simulink model "rigLoggerMultipacket"  (R2012b)
settings: Solver=FixedStepDiscrete  StartTime=0.0  StopTime=10.0  FixedStep=0.001  RelTol=1e-3
undefined symbols (not defined in the file): macaddr, modelConstants
libraries: simulink x42, xpcethernetlib x29, xpcnetworkbufferlib x15, xpcutilitieslib x14, dspswit3 x14, dspmtrx3 x14, Lib_FileLoggerMultipacket x1
(part 4 of 5)

== matlab function rigLoggerMultipacket/Neural2 Data & Format1/File Logger Format/File Logger Multipacket/Send Multipacket UDP/For Iterator
Subsystem/MATLAB Function ==
  data: data input uint8; numPackets input uint16 size=1; idxPacket input uint16 size=1; packetIP output uint8; lengthIP output uint16 size=1; sourceIP input uint8 size=4; sourcePort input uint16 size=1; destIP input uint8 size=4; destPort input uint16; datagramId input; prependHeader input
function [packetIP, lengthIP] = buildSubPacket(data, numPackets, idxPacket, sourceIP, sourcePort, destIP, destPort, datagramId, prependHeader)
%#codegen
% Creates a single UDP/IP packet that transmits one fragment of a possibly
% multi-fragment set of IP packets carrying the payload in data. idxPacket
% is the index of the fragment to send (1-indexed), out of num packets
% total fragments.
%
% Inputs:  
%   data : uint8 Nx1 or 1xN packet data vectors
%   numPackets, idxPacket : uint16 scalars
%   sourceIP, destIP : 1x4 uint8 of the IP (in address order)
%   sourcePort, destPort : uint16 port numbers
%   datagramId : uint16 scalar, unique id for this set of packets, for this timestep
%    that is used by the receiving IP stack to reassemble fragments
%   prependHeader : uint8 flag determining whether to prepend a 4 byte
%     header containing a 2 byte data length (excluding the header) and a 2
%     byte checksum (sum of bytes modulo 65536) of the data (excluding the 
%     header)
%
% Outputs:
%   packetIP : uint8 1500x1 IP packet to be passed into Create Ethernet
%     Packet block
%   lengthIP : uint16 scalar indicating the total length of packetIP
%     utilized, guaranteed to be even
% 
% Dan O'Shea, Paul Nuyujukian, Vikash Gilja
%

%% Initialize and return early if empty
packetIP = zeros(1500, 1, 'uint8');
lengthIP = uint16(0);

dataLength = numel(data);
if dataLength == 0
    return;
end

%% Build UDP subpacket

packetUDP = zeros(1480, 1, 'uint8');

% 1472 bytes per fragment
bytesPerFragment = uint16(1480);
headerUdpLength = uint16(8);
if prependHeader
    % 6 byte header on first packet containing '#u', 2 byte length, 2 byte checksum
    headerPreLength = uint16(4);
else
    headerPreLength = uint16(0);
end

headerLength = headerPreLength + headerUdpLength;

fragment = zeros(bytesPerFragment, 1, 'uint8');

% slice out the portion of data that goes in this packet
if idxPacket == 1
    byteStart = uint16(1);
    bytesThisFragment = bytesPerFragment - headerLength;
else
    % the first packet only graps 1480-8 bytes
    byteStart = uint16((idxPacket-uint16(1)) * bytesPerFragment - headerLength + uint16(1));
    bytesThisFragment = bytesPerFragment;
end

if byteStart > numel(data)
    % shouldn't happen, means idxPacket was too high for data
    return;
end
byteEnd = byteStart + bytesThisFragment - uint16(1);
% truncate fragment to data length
if byteEnd > numel(data)
    byteEnd = uint16(numel(data));
end
bytesThisFragment = byteEnd - byteStart + 1;

fragment(1:bytesThisFragment) = data(byteStart : byteEnd);

if idxPacket == 1
    if prependHeader
        headerPre = zeros(headerPreLength, 1, 'uint8');
        % 2 byte length
        headerPre(1:2) = typecast(uint16(numel(data)), 'uint8');
        % 2 byte modular checksum
        checksum = uint16(mod(sum(uint32(fragment)), uint32(65536)));
        headerPre(3:4) = typecast(checksum, 'uint8');
    else
        headerPre = [];
    end
        
    % include 8 byte udp header
    headerUdp = zeros(8, 1, 'uint8');
    FFFF = uint16(hex2dec('FFFF'));
    protocol = uint8(hex2dec('11'));
    length_BE = (typecast(uint16(numel(data)) + headerLength, 'uint8')); % flip to big endian
    length_BE = length_BE(end:-1:1);
    sourcePort_BE = (typecast(sourcePort, 'uint8'));
    sourcePort_BE = sourcePort_BE(end:-1:1);
    destPort_BE   = (typecast(destPort,   'uint8'));
    destPort_BE = destPort_BE(end:-1:1);
    headerUdp(1:8) = [sourcePort_BE destPort_BE length_BE uint8([0 0])];
    pseudoHeader = [sourceIP' destIP' uint8(0) protocol length_BE];
    
    if prependHeader
        % include 4 byte header in checksum
        if floor(double(numel(data)) / 2.0) ~= double(numel(data)) / 2.0
            % data is odd length, pad with zero byte
            checksumUdp = FFFF - uint16(mod( uint32(sum( typecast([pseudoHeader headerUdp' headerPre' data(:)' uint8(0)], 'uint16') )), uint32(FFFF) ));
        else
            checksumUdp = FFFF - uint16(mod( uint32(sum( typecast([pseudoHeader headerUdp' headerPre' data(:)'], 'uint16') )), uint32(FFFF) ));
        end
    else
        if floor(double(numel(data)) / 2.0) ~= double(numel(data)) / 2.0
            % data is odd length, pad with zero byte
            checksumUdp = FFFF - uint16(mod( uint32(sum( typecast([pseudoHeader headerUdp' data(:)' uint8(0)], 'uint16') )), uint32(FFFF) ));
        else
            checksumUdp = FFFF - uint16(mod( uint32(sum( typecast([pseudoHeader headerUdp' data(:)'], 'uint16') )), uint32(FFFF) ));
        end
    end
    headerUdp(7:8) = typecast(checksumUdp, 'uint8');

    % include custom 4 byte custom header with length and checksum
    if prependHeader
        lengthUDP = uint16(numel(headerUdp) + numel(headerPre) + bytesThisFragment);
        packetUDP(1:lengthUDP) = [headerUdp; headerPre; fragment(1:bytesThisFragment)];
    else
        % no header
        lengthUDP = uint16(numel(headerUdp) + bytesThisFragment);
        packetUDP(1:lengthUDP) = [headerUdp; fragment(1:bytesThisFragment)];
    end
else
    lengthUDP = uint16(bytesThisFragment);
    packetUDP(1:lengthUDP) = fragment(1:bytesThisFragment);
end

%% Build the fragment information that goes into IP header

% first 3 bits are 0, 1=DF, 2=More Fragments
% next 15 bits are length of fragment in bytes / 8
if idxPacket == 1
    fragmentWord = uint16(0);
else
    fragmentWord = (byteStart - uint16(1) + headerLength) / uint16(8);
end
if idxPacket < numPackets
    % set the more fragments bit
    fragmentWord = bitset(fragmentWord, 14);
end

% swap to big endian
fragmentBytes = typecast(fragmentWord, 'uint8')';
fragmentBytes = fragmentBytes([2;1]);

%% Build IP packet for this fragment

% make udp content length even
if floor(double(lengthUDP) / 2) ~= (double(lengthUDP) / 2)
    lengthUDP = lengthUDP + uint16(1);
end

% build IP header
lengthIP = lengthUDP + uint16(20);
version_IHL = uint8(69); % IPv4 and IP header length of 5
ToS = uint8(0); % no QOS on network

length_BE = (typecast(lengthIP, 'uint8')); % change to big endian
length_BE = length_BE(end:-1:1);

%ff = [ uint8(bin2dec('01000000')) 0 ]; % don't fragment packets
ff = fragmentBytes';
TTL = uint8(10); % ttl to 10 seconds/hops
protocol = uint8(hex2dec('11')); % UDP Protocol
headerIP = [ version_IHL ToS length_BE datagramId' ff TTL protocol 0 0 sourceIP' destIP'];

FFFF = uint16(hex2dec('FFFF'));
checksum = FFFF - uint16(mod( uint32(sum( typecast(headerIP, 'uint16') )), uint32(FFFF) ));
headerIP(11:12) = typecast(checksum, 'uint8');

% assemble the final packet
packetIP(1:lengthIP) = [ headerIP'; packetUDP(1:lengthUDP) ];

== matlab function rigLoggerMultipacket/DecoderC Data & Format1/File Logger Format/File Logger Multipacket/Send Multipacket UDP/For Iterator
Subsystem/MATLAB Function1 ==
  data: idx input; vec output; in input
function vec = storeInVector(idx, in)
%#codegen

nPacketsMax = 15;

persistent pVec;
if isempty(pVec) || idx == 1
    pVec = repmat(in*0, nPacketsMax, 1);
end
if idx >= 1 && idx <= nPacketsMax
    pVec(idx) = in;
end

vec = pVec;

== matlab function rigLoggerMultipacket/DecoderC Data & Format1/File Logger Format/File Logger Multipacket/Send Multipacket UDP/MATLAB Function ==
  data: in input; numPackets output uint16 size=1; prependHeader input
function numPackets = computeNumPackets(in, prependHeader)
%#codegen

% Assuming 1500 MTU, 1480 bytes per IP packet
% 8 bytes in udp header + 4 bytes in custom header if used, but only on the
% first fragment sent
if prependHeader
    headerLength = 8 + 6;
else
    headerLength = 8;
end
numPackets = uint16(ceil((double(numel(in))+headerLength) / 1480));

== matlab function rigLoggerMultipacket/DecoderC Data & Format1/File Logger Format/File Logger Multipacket/Send Multipacket UDP/MATLAB Function1 ==
  data: transmitId input uint8 size=1; datagramId output uint8 size=2
function datagramId = getDatagramId(transmitId)
%#codegen

% generates a unique id for this block, for this packet

persistent pId
if isempty(pId)
    pId = uint8(0);
else
    pId = pId + uint8(1);
end

datagramId = [transmitId; pId];

== matlab function rigLoggerMultipacket/DecoderD Data & Format1/File Logger Data/File Logger Multipacket/MATLAB Function1 ==
  data: u input; y output
function y = padFileName(u)

z = uint8(zeros(20, 1));

z(1:length(u)) = u;

y = z';

== matlab function rigLoggerMultipacket/DecoderD Data & Format1/File Logger Data/File Logger Multipacket/Send Multipacket UDP/For Iterator
Subsystem/MATLAB Function ==
  data: data input uint8; numPackets input uint16 size=1; idxPacket input uint16 size=1; packetIP output uint8; lengthIP output uint16 size=1; sourceIP input uint8 size=4; sourcePort input uint16 size=1; destIP input uint8 size=4; destPort input uint16; datagramId input; prependHeader input
function [packetIP, lengthIP] = buildSubPacket(data, numPackets, idxPacket, sourceIP, sourcePort, destIP, destPort, datagramId, prependHeader)
%#codegen
% Creates a single UDP/IP packet that transmits one fragment of a possibly
% multi-fragment set of IP packets carrying the payload in data. idxPacket
% is the index of the fragment to send (1-indexed), out of num packets
% total fragments.
%
% Inputs:  
%   data : uint8 Nx1 or 1xN packet data vectors
%   numPackets, idxPacket : uint16 scalars
%   sourceIP, destIP : 1x4 uint8 of the IP (in address order)
%   sourcePort, destPort : uint16 port numbers
%   datagramId : uint16 scalar, unique id for this set of packets, for this timestep
%    that is used by the receiving IP stack to reassemble fragments
%   prependHeader : uint8 flag determining whether to prepend a 4 byte
%     header containing a 2 byte data length (excluding the header) and a 2
%     byte checksum (sum of bytes modulo 65536) of the data (excluding the 
%     header)
%
% Outputs:
%   packetIP : uint8 1500x1 IP packet to be passed into Create Ethernet
%     Packet block
%   lengthIP : uint16 scalar indicating the total length of packetIP
%     utilized, guaranteed to be even
% 
% Dan O'Shea, Paul Nuyujukian, Vikash Gilja
%

%% Initialize and return early if empty
packetIP = zeros(1500, 1, 'uint8');
lengthIP = uint16(0);

dataLength = numel(data);
if dataLength == 0
    return;
end

%% Build UDP subpacket

packetUDP = zeros(1480, 1, 'uint8');

% 1472 bytes per fragment
bytesPerFragment = uint16(1480);
headerUdpLength = uint16(8);
if prependHeader
    % 6 byte header on first packet containing '#u', 2 byte length, 2 byte checksum
    headerPreLength = uint16(4);
else
    headerPreLength = uint16(0);
end

headerLength = headerPreLength + headerUdpLength;

fragment = zeros(bytesPerFragment, 1, 'uint8');

% slice out the portion of data that goes in this packet
if idxPacket == 1
    byteStart = uint16(1);
    bytesThisFragment = bytesPerFragment - headerLength;
else
    % the first packet only graps 1480-8 bytes
    byteStart = uint16((idxPacket-uint16(1)) * bytesPerFragment - headerLength + uint16(1));
    bytesThisFragment = bytesPerFragment;
end

if byteStart > numel(data)
    % shouldn't happen, means idxPacket was too high for data
    return;
end
byteEnd = byteStart + bytesThisFragment - uint16(1);
% truncate fragment to data length
if byteEnd > numel(data)
    byteEnd = uint16(numel(data));
end
bytesThisFragment = byteEnd - byteStart + 1;

fragment(1:bytesThisFragment) = data(byteStart : byteEnd);

if idxPacket == 1
    if prependHeader
        headerPre = zeros(headerPreLength, 1, 'uint8');
        % 2 byte length
        headerPre(1:2) = typecast(uint16(numel(data)), 'uint8');
        % 2 byte modular checksum
        checksum = uint16(mod(sum(uint32(fragment)), uint32(65536)));
        headerPre(3:4) = typecast(checksum, 'uint8');
    else
        headerPre = [];
    end
        
    % include 8 byte udp header
    headerUdp = zeros(8, 1, 'uint8');
    FFFF = uint16(hex2dec('FFFF'));
    protocol = uint8(hex2dec('11'));
    length_BE = (typecast(uint16(numel(data)) + headerLength, 'uint8')); % flip to big endian
    length_BE = length_BE(end:-1:1);
    sourcePort_BE = (typecast(sourcePort, 'uint8'));
    sourcePort_BE = sourcePort_BE(end:-1:1);
    destPort_BE   = (typecast(destPort,   'uint8'));
    destPort_BE = destPort_BE(end:-1:1);
    headerUdp(1:8) = [sourcePort_BE destPort_BE length_BE uint8([0 0])];
    pseudoHeader = [sourceIP' destIP' uint8(0) protocol length_BE];
    
    if prependHeader
        % include 4 byte header in checksum
        if floor(double(numel(data)) / 2.0) ~= double(numel(data)) / 2.0
            % data is odd length, pad with zero byte
            checksumUdp = FFFF - uint16(mod( uint32(sum( typecast([pseudoHeader headerUdp' headerPre' data(:)' uint8(0)], 'uint16') )), uint32(FFFF) ));
        else
            checksumUdp = FFFF - uint16(mod( uint32(sum( typecast([pseudoHeader headerUdp' headerPre' data(:)'], 'uint16') )), uint32(FFFF) ));
        end
    else
        if floor(double(numel(data)) / 2.0) ~= double(numel(data)) / 2.0
            % data is odd length, pad with zero byte
            checksumUdp = FFFF - uint16(mod( uint32(sum( typecast([pseudoHeader headerUdp' data(:)' uint8(0)], 'uint16') )), uint32(FFFF) ));
        else
            checksumUdp = FFFF - uint16(mod( uint32(sum( typecast([pseudoHeader headerUdp' data(:)'], 'uint16') )), uint32(FFFF) ));
        end
    end
    headerUdp(7:8) = typecast(checksumUdp, 'uint8');

    % include custom 4 byte custom header with length and checksum
    if prependHeader
        lengthUDP = uint16(numel(headerUdp) + numel(headerPre) + bytesThisFragment);
        packetUDP(1:lengthUDP) = [headerUdp; headerPre; fragment(1:bytesThisFragment)];
    else
        % no header
        lengthUDP = uint16(numel(headerUdp) + bytesThisFragment);
        packetUDP(1:lengthUDP) = [headerUdp; fragment(1:bytesThisFragment)];
    end
else
    lengthUDP = uint16(bytesThisFragment);
    packetUDP(1:lengthUDP) = fragment(1:bytesThisFragment);
end

%% Build the fragment information that goes into IP header

% first 3 bits are 0, 1=DF, 2=More Fragments
% next 15 bits are length of fragment in bytes / 8
if idxPacket == 1
    fragmentWord = uint16(0);
else
    fragmentWord = (byteStart - uint16(1) + headerLength) / uint16(8);
end
if idxPacket < numPackets
    % set the more fragments bit
    fragmentWord = bitset(fragmentWord, 14);
end

% swap to big endian
fragmentBytes = typecast(fragmentWord, 'uint8')';
fragmentBytes = fragmentBytes([2;1]);

%% Build IP packet for this fragment

% make udp content length even
if floor(double(lengthUDP) / 2) ~= (double(lengthUDP) / 2)
    lengthUDP = lengthUDP + uint16(1);
end

% build IP header
lengthIP = lengthUDP + uint16(20);
version_IHL = uint8(69); % IPv4 and IP header length of 5
ToS = uint8(0); % no QOS on network

length_BE = (typecast(lengthIP, 'uint8')); % change to big endian
length_BE = length_BE(end:-1:1);

%ff = [ uint8(bin2dec('01000000')) 0 ]; % don't fragment packets
ff = fragmentBytes';
TTL = uint8(10); % ttl to 10 seconds/hops
protocol = uint8(hex2dec('11')); % UDP Protocol
headerIP = [ version_IHL ToS length_BE datagramId' ff TTL protocol 0 0 sourceIP' destIP'];

FFFF = uint16(hex2dec('FFFF'));
checksum = FFFF - uint16(mod( uint32(sum( typecast(headerIP, 'uint16') )), uint32(FFFF) ));
headerIP(11:12) = typecast(checksum, 'uint8');

% assemble the final packet
packetIP(1:lengthIP) = [ headerIP'; packetUDP(1:lengthUDP) ];

== system rigLoggerMultipacket/Neural Data & Format1/File Logger Data/File Logger Multipacket/Send Multipacket UDP/For Iterator Subsystem ==
  Data : Inport  OutDataTypeStr=uint8
  Num Packets : Inport  Port=2  OutDataTypeStr=uint16  PortDimensions=1
  Datagram Id : Inport  Port=3  OutDataTypeStr=uint8  PortDimensions=2
  sourceIP : Inport  Port=4
  destIP : Inport  Port=5
  sourcePort : Inport  Port=6
  destPort : Inport  Port=7
  Constant1 : Constant  Value=uint8(prependHeader)  OutDataTypeStr=uint8
  "Create Ethernet Packet " : xpcethernetlib/Create Ethernet Packet   DstMac=destMac  EtherType=hex2dec('0800')
  DCT : DataTypeConversion  OutDataTypeStr=double
  Data Type Conversion : DataTypeConversion  OutDataTypeStr=uint16
  For Iterator : ForIterator  IterationSource=external  IterationVariableDataType=int16
  MATLAB Function : MATLAB Function  TreatAsAtomicUnit=on
  MATLAB Function1 : MATLAB Function  TreatAsAtomicUnit=on
  NB Vector : Outport
  wires:
  MATLAB Function1/1(vec) -> NB Vector/1
  "Create Ethernet Packet "/1 -> MATLAB Function1/2(in)
  Datagram Id/1 -> MATLAB Function/8(datagramId)
  sourceIP/1 -> MATLAB Function/4(sourceIP)
  destIP/1 -> MATLAB Function/6(destIP)
  destPort/1 -> MATLAB Function/7(destPort)
  DCT/1 -> "Create Ethernet Packet "/2
  MATLAB Function/1(packetIP) -> "Create Ethernet Packet "/1
  MATLAB Function/2(lengthIP) -> DCT/1
  Constant1/1 -> MATLAB Function/9(prependHeader)
  sourcePort/1 -> MATLAB Function/5(sourcePort)
  Data/1 -> MATLAB Function/1(data)
  Data Type Conversion/1 -> MATLAB Function1/1(idx), MATLAB Function/3(idxPacket)
  Num Packets/1 -> For Iterator/1, MATLAB Function/2(numPackets)
  For Iterator/1 -> Data Type Conversion/1

== system rigLoggerMultipacket/Neural Data & Format1/File Logger Format/File Logger Multipacket/Send Multipacket UDP/For Iterator Subsystem ==
  Data : Inport  OutDataTypeStr=uint8
  Num Packets : Inport  Port=2  OutDataTypeStr=uint16  PortDimensions=1
  Datagram Id : Inport  Port=3  OutDataTypeStr=uint8  PortDimensions=2
  sourceIP : Inport  Port=4
  destIP : Inport  Port=5
  sourcePort : Inport  Port=6
  destPort : Inport  Port=7
  Constant1 : Constant  Value=uint8(prependHeader)  OutDataTypeStr=uint8
  "Create Ethernet Packet " : xpcethernetlib/Create Ethernet Packet   DstMac=destMac  EtherType=hex2dec('0800')
  DCT : DataTypeConversion  OutDataTypeStr=double
  Data Type Conversion : DataTypeConversion  OutDataTypeStr=uint16
  For Iterator : ForIterator  IterationSource=external  IterationVariableDataType=int16
  MATLAB Function : MATLAB Function  TreatAsAtomicUnit=on
  MATLAB Function1 : MATLAB Function  TreatAsAtomicUnit=on
  NB Vector : Outport
  wires:
  MATLAB Function1/1(vec) -> NB Vector/1
  "Create Ethernet Packet "/1 -> MATLAB Function1/2(in)
  Datagram Id/1 -> MATLAB Function/8(datagramId)
  sourceIP/1 -> MATLAB Function/4(sourceIP)
  destIP/1 -> MATLAB Function/6(destIP)
  destPort/1 -> MATLAB Function/7(destPort)
  DCT/1 -> "Create Ethernet Packet "/2
  MATLAB Function/1(packetIP) -> "Create Ethernet Packet "/1
  MATLAB Function/2(lengthIP) -> DCT/1
  Constant1/1 -> MATLAB Function/9(prependHeader)
  sourcePort/1 -> MATLAB Function/5(sourcePort)
  Data/1 -> MATLAB Function/1(data)
  Data Type Conversion/1 -> MATLAB Function1/1(idx), MATLAB Function/3(idxPacket)
  Num Packets/1 -> For Iterator/1, MATLAB Function/2(numPackets)
  For Iterator/1 -> Data Type Conversion/1

== system rigLoggerMultipacket/Neural2 Data & Format1/File Logger Data/File Logger Multipacket/Send Multipacket UDP/For Iterator Subsystem ==
  Data : Inport  OutDataTypeStr=uint8
  Num Packets : Inport  Port=2  OutDataTypeStr=uint16  PortDimensions=1
  Datagram Id : Inport  Port=3  OutDataTypeStr=uint8  PortDimensions=2
  sourceIP : Inport  Port=4
  destIP : Inport  Port=5
  sourcePort : Inport  Port=6
  destPort : Inport  Port=7
  Constant1 : Constant  Value=uint8(prependHeader)  OutDataTypeStr=uint8
  "Create Ethernet Packet " : xpcethernetlib/Create Ethernet Packet   DstMac=destMac  EtherType=hex2dec('0800')
  DCT : DataTypeConversion  OutDataTypeStr=double
  Data Type Conversion : DataTypeConversion  OutDataTypeStr=uint16
  For Iterator : ForIterator  IterationSource=external  IterationVariableDataType=int16
  MATLAB Function : MATLAB Function  TreatAsAtomicUnit=on
  MATLAB Function1 : MATLAB Function  TreatAsAtomicUnit=on
  NB Vector : Outport
  wires:
  MATLAB Function1/1(vec) -> NB Vector/1
  "Create Ethernet Packet "/1 -> MATLAB Function1/2(in)
  Datagram Id/1 -> MATLAB Function/8(datagramId)
  sourceIP/1 -> MATLAB Function/4(sourceIP)
  destIP/1 -> MATLAB Function/6(destIP)
  destPort/1 -> MATLAB Function/7(destPort)
  DCT/1 -> "Create Ethernet Packet "/2
  MATLAB Function/1(packetIP) -> "Create Ethernet Packet "/1
  MATLAB Function/2(lengthIP) -> DCT/1
  Constant1/1 -> MATLAB Function/9(prependHeader)
  sourcePort/1 -> MATLAB Function/5(sourcePort)
  Data/1 -> MATLAB Function/1(data)
  Data Type Conversion/1 -> MATLAB Function1/1(idx), MATLAB Function/3(idxPacket)
  Num Packets/1 -> For Iterator/1, MATLAB Function/2(numPackets)
  For Iterator/1 -> Data Type Conversion/1

== system rigLoggerMultipacket/Neural2 Data & Format1/File Logger Format/File Logger Multipacket/Send Multipacket UDP/For Iterator Subsystem ==
  Data : Inport  OutDataTypeStr=uint8
  Num Packets : Inport  Port=2  OutDataTypeStr=uint16  PortDimensions=1
  Datagram Id : Inport  Port=3  OutDataTypeStr=uint8  PortDimensions=2
  sourceIP : Inport  Port=4
  destIP : Inport  Port=5
  sourcePort : Inport  Port=6
  destPort : Inport  Port=7
  Constant1 : Constant  Value=uint8(prependHeader)  OutDataTypeStr=uint8
  "Create Ethernet Packet " : xpcethernetlib/Create Ethernet Packet   DstMac=destMac  EtherType=hex2dec('0800')
  DCT : DataTypeConversion  OutDataTypeStr=double
  Data Type Conversion : DataTypeConversion  OutDataTypeStr=uint16
  For Iterator : ForIterator  IterationSource=external  IterationVariableDataType=int16
  MATLAB Function : MATLAB Function  TreatAsAtomicUnit=on
  MATLAB Function1 : MATLAB Function  TreatAsAtomicUnit=on
  NB Vector : Outport
  wires:
  MATLAB Function1/1(vec) -> NB Vector/1
  "Create Ethernet Packet "/1 -> MATLAB Function1/2(in)
  Datagram Id/1 -> MATLAB Function/8(datagramId)
  sourceIP/1 -> MATLAB Function/4(sourceIP)
  destIP/1 -> MATLAB Function/6(destIP)
  destPort/1 -> MATLAB Function/7(destPort)
  DCT/1 -> "Create Ethernet Packet "/2
  MATLAB Function/1(packetIP) -> "Create Ethernet Packet "/1
  MATLAB Function/2(lengthIP) -> DCT/1
  Constant1/1 -> MATLAB Function/9(prependHeader)
  sourcePort/1 -> MATLAB Function/5(sourcePort)
  Data/1 -> MATLAB Function/1(data)
  Data Type Conversion/1 -> MATLAB Function1/1(idx), MATLAB Function/3(idxPacket)
  Num Packets/1 -> For Iterator/1, MATLAB Function/2(numPackets)
  For Iterator/1 -> Data Type Conversion/1

== matlab function rigLoggerMultipacket/Task Details/File Logger Multipacket/MATLAB Function1 ==
  data: u input; y output
function y = padFileName(u)

z = uint8(zeros(20, 1));

z(1:length(u)) = u;

y = z';

== matlab function rigLoggerMultipacket/Task Details/File Logger Multipacket/Send Multipacket UDP/For Iterator Subsystem/MATLAB Function ==
  data: data input uint8; numPackets input uint16 size=1; idxPacket input uint16 size=1; packetIP output uint8; lengthIP output uint16 size=1; sourceIP input uint8 size=4; sourcePort input uint16 size=1; destIP input uint8 size=4; destPort input uint16; datagramId input; prependHeader input
function [packetIP, lengthIP] = buildSubPacket(data, numPackets, idxPacket, sourceIP, sourcePort, destIP, destPort, datagramId, prependHeader)
%#codegen
% Creates a single UDP/IP packet that transmits one fragment of a possibly
% multi-fragment set of IP packets carrying the payload in data. idxPacket
% is the index of the fragment to send (1-indexed), out of num packets
% total fragments.
%
% Inputs:  
%   data : uint8 Nx1 or 1xN packet data vectors
%   numPackets, idxPacket : uint16 scalars
%   sourceIP, destIP : 1x4 uint8 of the IP (in address order)
%   sourcePort, destPort : uint16 port numbers
%   datagramId : uint16 scalar, unique id for this set of packets, for this timestep
%    that is used by the receiving IP stack to reassemble fragments
%   prependHeader : uint8 flag determining whether to prepend a 4 byte
%     header containing a 2 byte data length (excluding the header) and a 2
%     byte checksum (sum of bytes modulo 65536) of the data (excluding the 
%     header)
%
% Outputs:
%   packetIP : uint8 1500x1 IP packet to be passed into Create Ethernet
%     Packet block
%   lengthIP : uint16 scalar indicating the total length of packetIP
%     utilized, guaranteed to be even
% 
% Dan O'Shea, Paul Nuyujukian, Vikash Gilja
%

%% Initialize and return early if empty
packetIP = zeros(1500, 1, 'uint8');
lengthIP = uint16(0);

dataLength = numel(data);
if dataLength == 0
    return;
end

%% Build UDP subpacket

packetUDP = zeros(1480, 1, 'uint8');

% 1472 bytes per fragment
bytesPerFragment = uint16(1480);
headerUdpLength = uint16(8);
if prependHeader
    % 6 byte header on first packet containing '#u', 2 byte length, 2 byte checksum
    headerPreLength = uint16(4);
else
    headerPreLength = uint16(0);
end

headerLength = headerPreLength + headerUdpLength;

fragment = zeros(bytesPerFragment, 1, 'uint8');

% slice out the portion of data that goes in this packet
if idxPacket == 1
    byteStart = uint16(1);
    bytesThisFragment = bytesPerFragment - headerLength;
else
    % the first packet only graps 1480-8 bytes
    byteStart = uint16((idxPacket-uint16(1)) * bytesPerFragment - headerLength + uint16(1));
    bytesThisFragment = bytesPerFragment;
end

if byteStart > numel(data)
    % shouldn't happen, means idxPacket was too high for data
    return;
end
byteEnd = byteStart + bytesThisFragment - uint16(1);
% truncate fragment to data length
if byteEnd > numel(data)
    byteEnd = uint16(numel(data));
end
bytesThisFragment = byteEnd - byteStart + 1;

fragment(1:bytesThisFragment) = data(byteStart : byteEnd);

if idxPacket == 1
    if prependHeader
        headerPre = zeros(headerPreLength, 1, 'uint8');
        % 2 byte length
        headerPre(1:2) = typecast(uint16(numel(data)), 'uint8');
        % 2 byte modular checksum
        checksum = uint16(mod(sum(uint32(fragment)), uint32(65536)));
        headerPre(3:4) = typecast(checksum, 'uint8');
    else
        headerPre = [];
    end
        
    % include 8 byte udp header
    headerUdp = zeros(8, 1, 'uint8');
    FFFF = uint16(hex2dec('FFFF'));
    protocol = uint8(hex2dec('11'));
    length_BE = (typecast(uint16(numel(data)) + headerLength, 'uint8')); % flip to big endian
    length_BE = length_BE(end:-1:1);
    sourcePort_BE = (typecast(sourcePort, 'uint8'));
    sourcePort_BE = sourcePort_BE(end:-1:1);
    destPort_BE   = (typecast(destPort,   'uint8'));
    destPort_BE = destPort_BE(end:-1:1);
    headerUdp(1:8) = [sourcePort_BE destPort_BE length_BE uint8([0 0])];
    pseudoHeader = [sourceIP' destIP' uint8(0) protocol length_BE];
    
    if prependHeader
        % include 4 byte header in checksum
        if floor(double(numel(data)) / 2.0) ~= double(numel(data)) / 2.0
            % data is odd length, pad with zero byte
            checksumUdp = FFFF - uint16(mod( uint32(sum( typecast([pseudoHeader headerUdp' headerPre' data(:)' uint8(0)], 'uint16') )), uint32(FFFF) ));
        else
            checksumUdp = FFFF - uint16(mod( uint32(sum( typecast([pseudoHeader headerUdp' headerPre' data(:)'], 'uint16') )), uint32(FFFF) ));
        end
    else
        if floor(double(numel(data)) / 2.0) ~= double(numel(data)) / 2.0
            % data is odd length, pad with zero byte
            checksumUdp = FFFF - uint16(mod( uint32(sum( typecast([pseudoHeader headerUdp' data(:)' uint8(0)], 'uint16') )), uint32(FFFF) ));
        else
            checksumUdp = FFFF - uint16(mod( uint32(sum( typecast([pseudoHeader headerUdp' data(:)'], 'uint16') )), uint32(FFFF) ));
        end
    end
    headerUdp(7:8) = typecast(checksumUdp, 'uint8');

    % include custom 4 byte custom header with length and checksum
    if prependHeader
        lengthUDP = uint16(numel(headerUdp) + numel(headerPre) + bytesThisFragment);
        packetUDP(1:lengthUDP) = [headerUdp; headerPre; fragment(1:bytesThisFragment)];
    else
        % no header
        lengthUDP = uint16(numel(headerUdp) + bytesThisFragment);
        packetUDP(1:lengthUDP) = [headerUdp; fragment(1:bytesThisFragment)];
    end
else
    lengthUDP = uint16(bytesThisFragment);
    packetUDP(1:lengthUDP) = fragment(1:bytesThisFragment);
end

%% Build the fragment information that goes into IP header

% first 3 bits are 0, 1=DF, 2=More Fragments
% next 15 bits are length of fragment in bytes / 8
if idxPacket == 1 && numPackets == 1
    fragmentWord = uint16(16384);
elseif idxPacket == 1
    fragmentWord = uint16(0);
else
    fragmentWord = (byteStart - uint16(1) + headerLength) / uint16(8);
end
if idxPacket < numPackets
    % set the more fragments bit
    fragmentWord = bitset(fragmentWord, 14);
end

% swap to big endian
fragmentBytes = typecast(fragmentWord, 'uint8')';
fragmentBytes = fragmentBytes([2;1]);

%% Build IP packet for this fragment

% make udp content length even
if floor(double(lengthUDP) / 2) ~= (double(lengthUDP) / 2)
    lengthUDP = lengthUDP + uint16(1);
end

% build IP header
lengthIP = lengthUDP + uint16(20);
version_IHL = uint8(69); % IPv4 and IP header length of 5
ToS = uint8(0); % no QOS on network

length_BE = (typecast(lengthIP, 'uint8')); % change to big endian
length_BE = length_BE(end:-1:1);

%ff = [ uint8(bin2dec('01000000')) 0 ]; % don't fragment packets
ff = fragmentBytes';
TTL = uint8(10); % ttl to 10 seconds/hops
protocol = uint8(hex2dec('11')); % UDP Protocol
headerIP = [ version_IHL ToS length_BE datagramId' ff TTL protocol 0 0 sourceIP' destIP'];

FFFF = uint16(hex2dec('FFFF'));
checksum = FFFF - uint16(mod( uint32(sum( typecast(headerIP, 'uint16') )), uint32(FFFF) ));
headerIP(11:12) = typecast(checksum, 'uint8');

% assemble the final packet
packetIP(1:lengthIP) = [ headerIP'; packetUDP(1:lengthUDP) ];

== matlab function rigLoggerMultipacket/Flush File Logger/Subsystem/Send Multipacket UDP/For Iterator Subsystem/MATLAB Function ==
  data: data input uint8; numPackets input uint16 size=1; idxPacket input uint16 size=1; packetIP output uint8; lengthIP output uint16 size=1; sourceIP input uint8 size=4; sourcePort input uint16 size=1; destIP input uint8 size=4; destPort input uint16; datagramId input; prependHeader input
function [packetIP, lengthIP] = buildSubPacket(data, numPackets, idxPacket, sourceIP, sourcePort, destIP, destPort, datagramId, prependHeader)
%#codegen
% Creates a single UDP/IP packet that transmits one fragment of a possibly
% multi-fragment set of IP packets carrying the payload in data. idxPacket
% is the index of the fragment to send (1-indexed), out of num packets
% total fragments.
%
% Inputs:  
%   data : uint8 Nx1 or 1xN packet data vectors
%   numPackets, idxPacket : uint16 scalars
%   sourceIP, destIP : 1x4 uint8 of the IP (in address order)
%   sourcePort, destPort : uint16 port numbers
%   datagramId : uint16 scalar, unique id for this set of packets, for this timestep
%    that is used by the receiving IP stack to reassemble fragments
%   prependHeader : uint8 flag determining whether to prepend a 4 byte
%     header containing a 2 byte data length (excluding the header) and a 2
%     byte checksum (sum of bytes modulo 65536) of the data (excluding the 
%     header)
%
% Outputs:
%   packetIP : uint8 1500x1 IP packet to be passed into Create Ethernet
%     Packet block
%   lengthIP : uint16 scalar indicating the total length of packetIP
%     utilized, guaranteed to be even
% 
% Dan O'Shea, Paul Nuyujukian, Vikash Gilja
%

%% Initialize and return early if empty
packetIP = zeros(1500, 1, 'uint8');
lengthIP = uint16(0);

dataLength = numel(data);
if dataLength == 0
    return;
end

%% Build UDP subpacket

packetUDP = zeros(1480, 1, 'uint8');

% 1472 bytes per fragment
bytesPerFragment = uint16(1480);
headerUdpLength = uint16(8);
if prependHeader
    % 6 byte header on first packet containing '#u', 2 byte length, 2 byte checksum
    headerPreLength = uint16(4);
else
    headerPreLength = uint16(0);
end

headerLength = headerPreLength + headerUdpLength;

fragment = zeros(bytesPerFragment, 1, 'uint8');

% slice out the portion of data that goes in this packet
if idxPacket == 1
    byteStart = uint16(1);
    bytesThisFragment = bytesPerFragment - headerLength;
else
    % the first packet only graps 1480-8 bytes
    byteStart = uint16((idxPacket-uint16(1)) * bytesPerFragment - headerLength + uint16(1));
    bytesThisFragment = bytesPerFragment;
end

if byteStart > numel(data)
    % shouldn't happen, means idxPacket was too high for data
    return;
end
byteEnd = byteStart + bytesThisFragment - uint16(1);
% truncate fragment to data length
if byteEnd > numel(data)
    byteEnd = uint16(numel(data));
end
bytesThisFragment = byteEnd - byteStart + 1;

fragment(1:bytesThisFragment) = data(byteStart : byteEnd);

if idxPacket == 1
    if prependHeader
        headerPre = zeros(headerPreLength, 1, 'uint8');
        % 2 byte length
        headerPre(1:2) = typecast(uint16(numel(data)), 'uint8');
        % 2 byte modular checksum
        checksum = uint16(mod(sum(uint32(fragment)), uint32(65536)));
        headerPre(3:4) = typecast(checksum, 'uint8');
    else
        headerPre = [];
    end
        
    % include 8 byte udp header
    headerUdp = zeros(8, 1, 'uint8');
    FFFF = uint16(hex2dec('FFFF'));
    protocol = uint8(hex2dec('11'));
    length_BE = (typecast(uint16(numel(data)) + headerLength, 'uint8')); % flip to big endian
    length_BE = length_BE(end:-1:1);
    sourcePort_BE = (typecast(sourcePort, 'uint8'));
    sourcePort_BE = sourcePort_BE(end:-1:1);
    destPort_BE   = (typecast(destPort,   'uint8'));
    destPort_BE = destPort_BE(end:-1:1);
    headerUdp(1:8) = [sourcePort_BE destPort_BE length_BE uint8([0 0])];
    pseudoHeader = [sourceIP' destIP' uint8(0) protocol length_BE];
    
    if prependHeader
        % include 4 byte header in checksum
        if floor(double(numel(data)) / 2.0) ~= double(numel(data)) / 2.0
            % data is odd length, pad with zero byte
            checksumUdp = FFFF - uint16(mod( uint32(sum( typecast([pseudoHeader headerUdp' headerPre' data(:)' uint8(0)], 'uint16') )), uint32(FFFF) ));
        else
            checksumUdp = FFFF - uint16(mod( uint32(sum( typecast([pseudoHeader headerUdp' headerPre' data(:)'], 'uint16') )), uint32(FFFF) ));
        end
    else
        if floor(double(numel(data)) / 2.0) ~= double(numel(data)) / 2.0
            % data is odd length, pad with zero byte
            checksumUdp = FFFF - uint16(mod( uint32(sum( typecast([pseudoHeader headerUdp' data(:)' uint8(0)], 'uint16') )), uint32(FFFF) ));
        else
            checksumUdp = FFFF - uint16(mod( uint32(sum( typecast([pseudoHeader headerUdp' data(:)'], 'uint16') )), uint32(FFFF) ));
        end
    end
    headerUdp(7:8) = typecast(checksumUdp, 'uint8');

    % include custom 4 byte custom header with length and checksum
    if prependHeader
        lengthUDP = uint16(numel(headerUdp) + numel(headerPre) + bytesThisFragment);
        packetUDP(1:lengthUDP) = [headerUdp; headerPre; fragment(1:bytesThisFragment)];
    else
        % no header
        lengthUDP = uint16(numel(headerUdp) + bytesThisFragment);
        packetUDP(1:lengthUDP) = [headerUdp; fragment(1:bytesThisFragment)];
    end
else
    lengthUDP = uint16(bytesThisFragment);
    packetUDP(1:lengthUDP) = fragment(1:bytesThisFragment);
end

%% Build the fragment information that goes into IP header

% first 3 bits are 0, 1=DF, 2=More Fragments
% next 15 bits are length of fragment in bytes / 8
if idxPacket == 1 && numPackets == 1
    fragmentWord = uint16(16384);
elseif idxPacket == 1
    fragmentWord = uint16(0);
else
    fragmentWord = (byteStart - uint16(1) + headerLength) / uint16(8);
end
if idxPacket < numPackets
    % set the more fragments bit
    fragmentWord = bitset(fragmentWord, 14);
end

% swap to big endian
fragmentBytes = typecast(fragmentWord, 'uint8')';
fragmentBytes = fragmentBytes([2;1]);

%% Build IP packet for this fragment

% make udp content length even
if floor(double(lengthUDP) / 2) ~= (double(lengthUDP) / 2)
    lengthUDP = lengthUDP + uint16(1);
end

% build IP header
lengthIP = lengthUDP + uint16(20);
version_IHL = uint8(69); % IPv4 and IP header length of 5
ToS = uint8(0); % no QOS on network

length_BE = (typecast(lengthIP, 'uint8')); % change to big endian
length_BE = length_BE(end:-1:1);

%ff = [ uint8(bin2dec('01000000')) 0 ]; % don't fragment packets
ff = fragmentBytes';
TTL = uint8(10); % ttl to 10 seconds/hops
protocol = uint8(hex2dec('11')); % UDP Protocol
headerIP = [ version_IHL ToS length_BE datagramId' ff TTL protocol 0 0 sourceIP' destIP'];

FFFF = uint16(hex2dec('FFFF'));
checksum = FFFF - uint16(mod( uint32(sum( typecast(headerIP, 'uint16') )), uint32(FFFF) ));
headerIP(11:12) = typecast(checksum, 'uint8');

% assemble the final packet
packetIP(1:lengthIP) = [ headerIP'; packetUDP(1:lengthUDP) ];

== matlab function rigLoggerMultipacket/Flush File Logger/Subsystem/Send Multipacket UDP/MATLAB Function ==
  data: in input; numPackets output uint16 size=1; prependHeader input
function numPackets = computeNumPackets(in, prependHeader)
%#codegen

% Assuming 1500 MTU, 1480 bytes per IP packet
% 8 bytes in udp header + 4 bytes in custom header if used, but only on the
% first fragment sent
if prependHeader
    headerLength = 8 + 6;
else
    headerLength = 8;
end
numPackets = uint16(ceil((double(numel(in))+headerLength) / 1480));

== matlab function rigLoggerMultipacket/Task Details/File Logger Multipacket/Send Multipacket UDP/For Iterator Subsystem/MATLAB Function1 ==
  data: idx input; vec output; in input
function vec = storeInVector(idx, in)
%#codegen

nPacketsMax = 15;

persistent pVec;
if isempty(pVec) || idx == 1
    pVec = repmat(in*0, nPacketsMax, 1);
end
if idx >= 1 && idx <= nPacketsMax
    pVec(idx) = in;
end

vec = pVec;

== matlab function rigLoggerMultipacket/Task Details/File Logger Multipacket/Send Multipacket UDP/MATLAB Function ==
  data: in input; numPackets output uint16 size=1; prependHeader input
function numPackets = computeNumPackets(in, prependHeader)
%#codegen

% Assuming 1500 MTU, 1480 bytes per IP packet
% 8 bytes in udp header + 4 bytes in custom header if used, but only on the
% first fragment sent
if prependHeader
    headerLength = 8 + 6;
else
    headerLength = 8;
end
numPackets = uint16(ceil((double(numel(in))+headerLength) / 1480));

== matlab function rigLoggerMultipacket/Task Details/File Logger Multipacket/Send Multipacket UDP/MATLAB Function1 ==
  data: transmitId input uint8 size=1; datagramId output uint8 size=2
function datagramId = getDatagramId(transmitId)
%#codegen

% generates a unique id for this block, for this packet

persistent pId
if isempty(pId)
    pId = uint8(0);
else
    pId = pId + uint8(1);
end

datagramId = [transmitId; pId];

== matlab function rigLoggerMultipacket/Flush File Logger/Subsystem/Send Multipacket UDP/MATLAB Function1 ==
  data: transmitId input uint8 size=1; datagramId output uint8 size=2
function datagramId = getDatagramId(transmitId)
%#codegen

% generates a unique id for this block, for this packet

persistent pId
if isempty(pId)
    pId = uint8(0);
else
    pId = pId + uint8(1);
end

datagramId = [transmitId; pId];

== matlab function rigLoggerMultipacket/Flush File Logger/Subsystem/Send Multipacket UDP/For Iterator Subsystem/MATLAB Function1 ==
  data: idx input; vec output; in input
function vec = storeInVector(idx, in)
%#codegen

nPacketsMax = 15;

persistent pVec;
if isempty(pVec) || idx == 1
    pVec = repmat(in*0, nPacketsMax, 1);
end
if idx >= 1 && idx <= nPacketsMax
    pVec(idx) = in;
end

vec = pVec;

== matlab function rigLoggerMultipacket/Discrete Data & Format/File Logger Data/File Logger Multipacket/MATLAB Function1 ==
  data: u input; y output
function y = padFileName(u)

z = uint8(zeros(20, 1));

z(1:length(u)) = u;

y = z';

== matlab function rigLoggerMultipacket/Discrete Data & Format/File Logger Data/File Logger Multipacket/Send Multipacket UDP/For Iterator Subsystem/MATLAB Function ==
  data: data input uint8; numPackets input uint16 size=1; idxPacket input uint16 size=1; packetIP output uint8; lengthIP output uint16 size=1; sourceIP input uint8 size=4; sourcePort input uint16 size=1; destIP input uint8 size=4; destPort input uint16; datagramId input; prependHeader input
function [packetIP, lengthIP] = buildSubPacket(data, numPackets, idxPacket, sourceIP, sourcePort, destIP, destPort, datagramId, prependHeader)
%#codegen
% Creates a single UDP/IP packet that transmits one fragment of a possibly
% multi-fragment set of IP packets carrying the payload in data. idxPacket
% is the index of the fragment to send (1-indexed), out of num packets
% total fragments.
%
% Inputs:  
%   data : uint8 Nx1 or 1xN packet data vectors
%   numPackets, idxPacket : uint16 scalars
%   sourceIP, destIP : 1x4 uint8 of the IP (in address order)
%   sourcePort, destPort : uint16 port numbers
%   datagramId : uint16 scalar, unique id for this set of packets, for this timestep
%    that is used by the receiving IP stack to reassemble fragments
%   prependHeader : uint8 flag determining whether to prepend a 4 byte
%     header containing a 2 byte data length (excluding the header) and a 2
%     byte checksum (sum of bytes modulo 65536) of the data (excluding the 
%     header)
%
% Outputs:
%   packetIP : uint8 1500x1 IP packet to be passed into Create Ethernet
%     Packet block
%   lengthIP : uint16 scalar indicating the total length of packetIP
%     utilized, guaranteed to be even
% 
% Dan O'Shea, Paul Nuyujukian, Vikash Gilja
%

%% Initialize and return early if empty
packetIP = zeros(1500, 1, 'uint8');
lengthIP = uint16(0);

dataLength = numel(data);
if dataLength == 0
    return;
end

%% Build UDP subpacket

packetUDP = zeros(1480, 1, 'uint8');

% 1472 bytes per fragment
bytesPerFragment = uint16(1480);
headerUdpLength = uint16(8);
if prependHeader
    % 6 byte header on first packet containing '#u', 2 byte length, 2 byte checksum
    headerPreLength = uint16(4);
else
    headerPreLength = uint16(0);
end

headerLength = headerPreLength + headerUdpLength;

fragment = zeros(bytesPerFragment, 1, 'uint8');

% slice out the portion of data that goes in this packet
if idxPacket == 1
    byteStart = uint16(1);
    bytesThisFragment = bytesPerFragment - headerLength;
else
    % the first packet only graps 1480-8 bytes
    byteStart = uint16((idxPacket-uint16(1)) * bytesPerFragment - headerLength + uint16(1));
    bytesThisFragment = bytesPerFragment;
end

if byteStart > numel(data)
    % shouldn't happen, means idxPacket was too high for data
    return;
end
byteEnd = byteStart + bytesThisFragment - uint16(1);
% truncate fragment to data length
if byteEnd > numel(data)
    byteEnd = uint16(numel(data));
end
bytesThisFragment = byteEnd - byteStart + 1;

fragment(1:bytesThisFragment) = data(byteStart : byteEnd);

if idxPacket == 1
    if prependHeader
        headerPre = zeros(headerPreLength, 1, 'uint8');
        % 2 byte length
        headerPre(1:2) = typecast(uint16(numel(data)), 'uint8');
        % 2 byte modular checksum
        checksum = uint16(mod(sum(uint32(fragment)), uint32(65536)));
        headerPre(3:4) = typecast(checksum, 'uint8');
    else
        headerPre = [];
    end
        
    % include 8 byte udp header
    headerUdp = zeros(8, 1, 'uint8');
    FFFF = uint16(hex2dec('FFFF'));
    protocol = uint8(hex2dec('11'));
    length_BE = (typecast(uint16(numel(data)) + headerLength, 'uint8')); % flip to big endian
    length_BE = length_BE(end:-1:1);
    sourcePort_BE = (typecast(sourcePort, 'uint8'));
    sourcePort_BE = sourcePort_BE(end:-1:1);
    destPort_BE   = (typecast(destPort,   'uint8'));
    destPort_BE = destPort_BE(end:-1:1);
    headerUdp(1:8) = [sourcePort_BE destPort_BE length_BE uint8([0 0])];
    pseudoHeader = [sourceIP' destIP' uint8(0) protocol length_BE];
    
    if prependHeader
        % include 4 byte header in checksum
        if floor(double(numel(data)) / 2.0) ~= double(numel(data)) / 2.0
            % data is odd length, pad with zero byte
            checksumUdp = FFFF - uint16(mod( uint32(sum( typecast([pseudoHeader headerUdp' headerPre' data(:)' uint8(0)], 'uint16') )), uint32(FFFF) ));
        else
            checksumUdp = FFFF - uint16(mod( uint32(sum( typecast([pseudoHeader headerUdp' headerPre' data(:)'], 'uint16') )), uint32(FFFF) ));
        end
    else
        if floor(double(numel(data)) / 2.0) ~= double(numel(data)) / 2.0
            % data is odd length, pad with zero byte
            checksumUdp = FFFF - uint16(mod( uint32(sum( typecast([pseudoHeader headerUdp' data(:)' uint8(0)], 'uint16') )), uint32(FFFF) ));
        else
            checksumUdp = FFFF - uint16(mod( uint32(sum( typecast([pseudoHeader headerUdp' data(:)'], 'uint16') )), uint32(FFFF) ));
        end
    end
    headerUdp(7:8) = typecast(checksumUdp, 'uint8');

    % include custom 4 byte custom header with length and checksum
    if prependHeader
        lengthUDP = uint16(numel(headerUdp) + numel(headerPre) + bytesThisFragment);
        packetUDP(1:lengthUDP) = [headerUdp; headerPre; fragment(1:bytesThisFragment)];
    else
        % no header
        lengthUDP = uint16(numel(headerUdp) + bytesThisFragment);
        packetUDP(1:lengthUDP) = [headerUdp; fragment(1:bytesThisFragment)];
    end
else
    lengthUDP = uint16(bytesThisFragment);
    packetUDP(1:lengthUDP) = fragment(1:bytesThisFragment);
end

%% Build the fragment information that goes into IP header

% first 3 bits are 0, 1=DF, 2=More Fragments
% next 15 bits are length of fragment in bytes / 8
if idxPacket == 1 && numPackets == 1
    fragmentWord = uint16(16384);
elseif idxPacket == 1
    fragmentWord = uint16(0);
else
    fragmentWord = (byteStart - uint16(1) + headerLength) / uint16(8);
end
if idxPacket < numPackets
    % set the more fragments bit
    fragmentWord = bitset(fragmentWord, 14);
end

% swap to big endian
fragmentBytes = typecast(fragmentWord, 'uint8')';
fragmentBytes = fragmentBytes([2;1]);

%% Build IP packet for this fragment

% make udp content length even
if floor(double(lengthUDP) / 2) ~= (double(lengthUDP) / 2)
    lengthUDP = lengthUDP + uint16(1);
end

% build IP header
lengthIP = lengthUDP + uint16(20);
version_IHL = uint8(69); % IPv4 and IP header length of 5
ToS = uint8(0); % no QOS on network

length_BE = (typecast(lengthIP, 'uint8')); % change to big endian
length_BE = length_BE(end:-1:1);

%ff = [ uint8(bin2dec('01000000')) 0 ]; % don't fragment packets
ff = fragmentBytes';
TTL = uint8(10); % ttl to 10 seconds/hops
protocol = uint8(hex2dec('11')); % UDP Protocol
headerIP = [ version_IHL ToS length_BE datagramId' ff TTL protocol 0 0 sourceIP' destIP'];

FFFF = uint16(hex2dec('FFFF'));
checksum = FFFF - uint16(mod( uint32(sum( typecast(headerIP, 'uint16') )), uint32(FFFF) ));
headerIP(11:12) = typecast(checksum, 'uint8');

% assemble the final packet
packetIP(1:lengthIP) = [ headerIP'; packetUDP(1:lengthUDP) ];

== matlab function rigLoggerMultipacket/Discrete Data & Format/File Logger Data/File Logger Multipacket/Send Multipacket UDP/For Iterator Subsystem/MATLAB Function1 ==
  data: idx input; vec output; in input
function vec = storeInVector(idx, in)
%#codegen

nPacketsMax = 15;

persistent pVec;
if isempty(pVec) || idx == 1
    pVec = repmat(in*0, nPacketsMax, 1);
end
if idx >= 1 && idx <= nPacketsMax
    pVec(idx) = in;
end

vec = pVec;

== matlab function rigLoggerMultipacket/Discrete Data & Format/File Logger Data/File Logger Multipacket/Send Multipacket UDP/MATLAB Function ==
  data: in input; numPackets output uint16 size=1; prependHeader input
function numPackets = computeNumPackets(in, prependHeader)
%#codegen

% Assuming 1500 MTU, 1480 bytes per IP packet
% 8 bytes in udp header + 4 bytes in custom header if used, but only on the
% first fragment sent
if prependHeader
    headerLength = 8 + 6;
else
    headerLength = 8;
end
numPackets = uint16(ceil((double(numel(in))+headerLength) / 1480));

== matlab function rigLoggerMultipacket/Discrete Data & Format/File Logger Data/File Logger Multipacket/Send Multipacket UDP/MATLAB Function1 ==
  data: transmitId input uint8 size=1; datagramId output uint8 size=2
function datagramId = getDatagramId(transmitId)
%#codegen

% generates a unique id for this block, for this packet

persistent pId
if isempty(pId)
    pId = uint8(0);
else
    pId = pId + uint8(1);
end

datagramId = [transmitId; pId];

== matlab function rigLoggerMultipacket/Discrete Data & Format/File Logger Format/File Logger Multipacket/MATLAB Function1 ==
  data: u input; y output
function y = padFileName(u)

z = uint8(zeros(20, 1));

z(1:length(u)) = u;

y = z';
